simulink model "FullControllerPartCAgain"  (R2012b)
settings: Solver=ode45  StartTime=0.0  StopTime=20.0  RelTol=1e-3
settings Model: Creator=Jake  LastModifiedBy=Jake

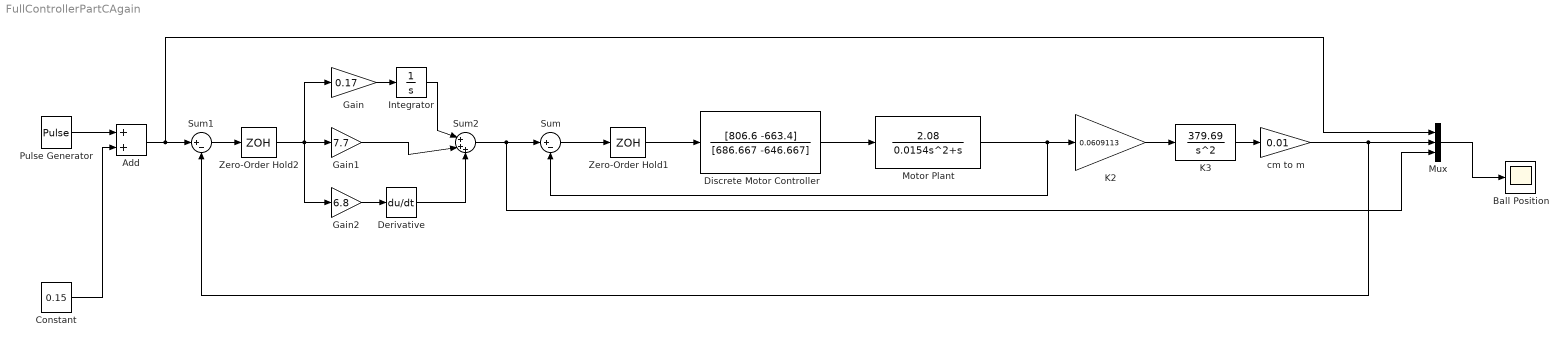
== system FullControllerPartCAgain ==
  Add : Sum
  Ball Position : Scope
      settings: TimeRange=50  YMin=-2500000000  YMax=47500000000  MaxDataPoints=500000
  Constant : Constant  Value=0.15
  Derivative : Derivative
  Discrete Motor Controller : DiscreteFilter  Numerator=[806.6 -663.4]  Denominator=[686.667 -646.667]
  Gain : Gain  Gain=0.17
  Gain1 : Gain  Gain=7.7
  Gain2 : Gain  Gain=6.8
  Integrator : Integrator
  "K2 " : Gain  Gain=0.0609113
  K3 : TransferFcn  Numerator=[379.69]  Denominator=[1 0 0]
  Motor Plant : TransferFcn  Numerator=[2.08]  Denominator=[0.0154 1 0]
  Mux : Mux  Inputs=3
  Pulse Generator : DiscretePulseGenerator  PulseType=Time based  Amplitude=0.03  Period=50  PulseWidth=50
  Sum : Sum  Inputs=|+-
  Sum1 : Sum  Inputs=|+-
  Sum2 : Sum  Inputs=|+++
  Zero-Order Hold1 : ZeroOrderHold  SampleTime=0.003
  Zero-Order Hold2 : ZeroOrderHold  SampleTime=0.003
  cm to m : Gain  Gain=0.01
  wires:
  Motor Plant/1 -> "K2 "/1, Sum/2
  "K2 "/1 -> K3/1
  Zero-Order Hold1/1 -> Discrete Motor Controller/1
  Pulse Generator/1 -> Add/1
  Constant/1 -> Add/2
  Add/1 -> Mux/1, Sum1/1
  Mux/1 -> Ball Position/1
  Discrete Motor Controller/1 -> Motor Plant/1
  Sum/1 -> Zero-Order Hold1/1
  K3/1 -> cm to m/1
  cm to m/1 -> Sum1/2, Mux/2
  Gain/1 -> Integrator/1
  Gain2/1 -> Derivative/1
  Sum2/1 -> Mux/3, Sum/1
  Gain1/1 -> Sum2/2
  Integrator/1 -> Sum2/1
  Derivative/1 -> Sum2/3
  Zero-Order Hold2/1 -> Gain2/1, Gain/1, Gain1/1
  Sum1/1 -> Zero-Order Hold2/1
